simulink model "Enum"  (R2021b)
settings: Solver=VariableStepAuto  StartTime=0.0  StopTime=10.0  RelTol=1e-3
undefined symbols (not defined in the file or in its folder): Number
libraries: simulink x1
settings Model: Creator=fady  LastModifiedBy=fady

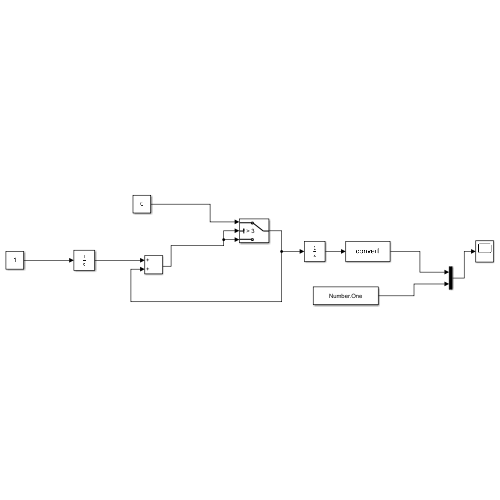
[thumbnail: Simulink's stored preview of the top-level diagram]
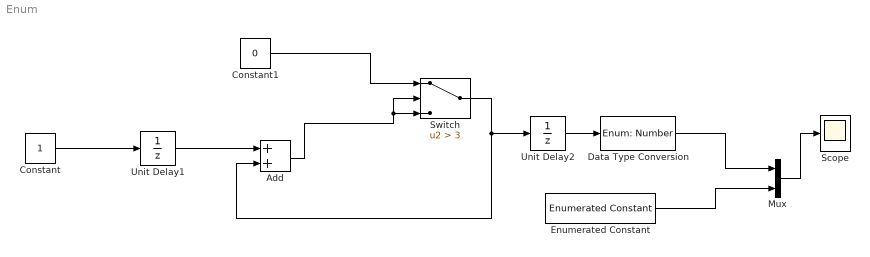
== system Enum ==
  Add : Sum  OutDataTypeStr=int32
  Constant : Constant  OutDataTypeStr=int32
  Constant1 : Constant  Value=0  OutDataTypeStr=int32
  Data Type Conversion : DataTypeConversion  OutDataTypeStr=Enum: Number
  Enumerated Constant : simulink/Sources/Enumerated Constant  OutDataTypeStr=Enum: Number  Value=Number.One  SampleTime=inf
  Mux : Mux  Inputs=2
  Scope : Scope
  Switch : Switch  Criteria=u2 > Threshold  Threshold=3  OutDataTypeStr=int32
  Unit Delay1 : UnitDelay  SampleTime=-1  HasFrameUpgradeWarning=on
  Unit Delay2 : UnitDelay  SampleTime=-1  HasFrameUpgradeWarning=on
  wires:
  Add/1 -> Switch/3, Switch/2
  Constant1/1 -> Switch/1
  Constant/1 -> Unit Delay1/1
  Unit Delay1/1 -> Add/1
  Switch/1 -> Add/2, Unit Delay2/1
  Unit Delay2/1 -> Data Type Conversion/1
  Mux/1 -> Scope/1
  Data Type Conversion/1 -> Mux/1
  Enumerated Constant/1 -> Mux/2
